simulink model "simulation_commande_adaptative_amine"  (R2020a)
settings: Solver=VariableStepAuto  StartTime=0.0  StopTime=100  RelTol=1e-3
settings Model: Creator=amine  LastModifiedBy=lenovo

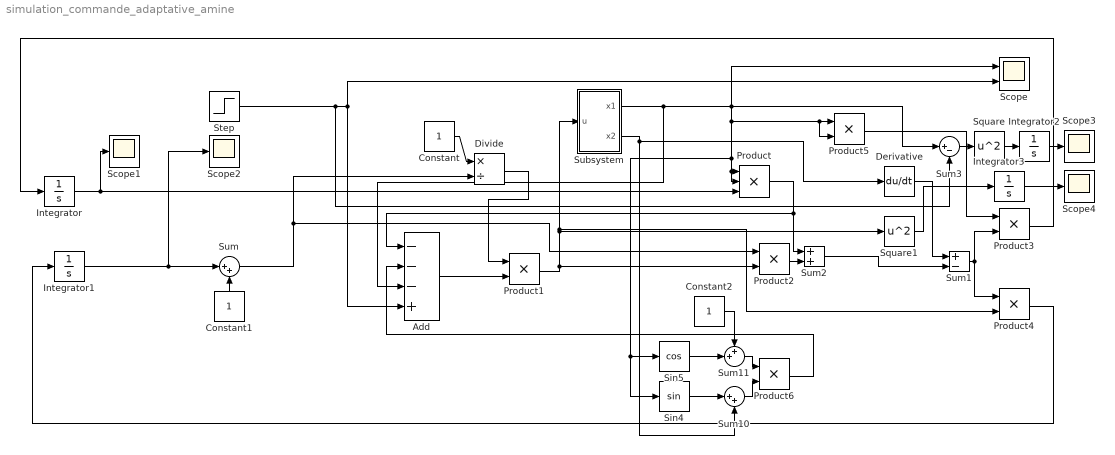
== system simulation_commande_adaptative_amine ==
  Add : Sum  Inputs=---+
  Constant : Constant
  Constant1 : Constant
  Constant2 : Constant
  Derivative : Derivative
  Divide : Product  Inputs=*/
  Integrator{,1..3} (4 alike) : Integrator
  Product : Product  Inputs=3
  Product{1..6} (6 alike) : Product
  Scope : Scope  NumInputPorts=2
  Scope{1..4} (4 alike) : Scope
  Sin4 : Trigonometry
  Sin5 : Trigonometry  Operator=cos
  Square : Math  Operator=square  SaturateOnIntegerOverflow=on
  Square1 : Math  Operator=square  SaturateOnIntegerOverflow=on
  Step : Step  Time=0  SampleTime=0
  Subsystem : Subsystem
  Sum : Sum  Inputs=|++
  Sum1 : Sum  Inputs=+-
  Sum10 : Sum  Inputs=|++
  Sum11 : Sum  Inputs=++|
  Sum2 : Sum
  Sum3 : Sum  Inputs=|+-
  wires:
  Sin5/1 -> Sum11/2
  Sum10/1 -> Product6/2
  Subsystem/2(x2) -> Derivative/1, Sum10/2
  Product/1 -> Sum2/1, Add/1
  Sin4/1 -> Sum10/1
  Product6/1 -> Add/2
  Constant2/1 -> Sum11/1
  Subsystem/1(x1) -> Add/3, Sum3/1, Product5/2, Product5/1, Product/2, Product/1, Sin5/1, Sin4/1, Scope/1
  Sum11/1 -> Product6/1
  Add/1 -> Product1/2
  Step/1 -> Sum3/2, Scope/2, Add/4
  Product1/1 -> Product2/2, Subsystem/1(u), Product4/2, Square1/1
  Constant/1 -> Divide/1
  Sum/1 -> Product2/1, Divide/2
  Constant1/1 -> Sum/2
  Integrator1/1 -> Scope2/1, Sum/1
  Divide/1 -> Product1/1
  Integrator/1 -> Scope1/1, Product/3
  Derivative/1 -> Sum1/1
  Product2/1 -> Sum2/2
  Sum2/1 -> Sum1/2
  Sum1/1 -> Product3/2, Product4/1
  Product5/1 -> Product3/1
  Product3/1 -> Integrator/1
  Product4/1 -> Integrator1/1
  Integrator2/1 -> Scope3/1
  Integrator3/1 -> Scope4/1
  Sum3/1 -> Square/1
  Square/1 -> Integrator2/1
  Square1/1 -> Integrator3/1

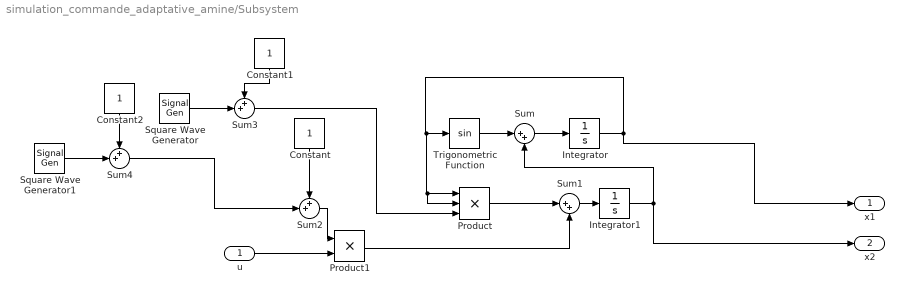
== system simulation_commande_adaptative_amine/Subsystem ==
  u : Inport
  Constant : Constant
  Constant1 : Constant
  Constant2 : Constant
  Integrator : Integrator
  Integrator1 : Integrator
  Product : Product  Inputs=3
  Product1 : Product
  Square Wave Generator : SignalGenerator  WaveForm=square  Amplitude=0.2  Frequency=0.05
  Square Wave Generator1 : SignalGenerator  WaveForm=square  Amplitude=0.2  Frequency=0.05
  Sum : Sum  Inputs=|++
  Sum1 : Sum  Inputs=|++
  Sum2 : Sum  Inputs=++|
  Sum3 : Sum  Inputs=++|
  Sum4 : Sum  Inputs=++|
  Trigonometric Function : Trigonometry
  x1 : Outport
  x2 : Outport  Port=2
  wires:
  Sum1/1 -> Integrator1/1
  Product/1 -> Sum1/1
  Integrator1/1 -> Sum/2, x2/1
  Trigonometric Function/1 -> Sum/1
  Integrator/1 -> Product/2, Product/1, Trigonometric Function/1, x1/1
  Sum/1 -> Integrator/1
  u/1 -> Product1/2
  Product1/1 -> Sum1/2
  Constant/1 -> Sum2/1
  Sum4/1 -> Sum2/2
  Sum2/1 -> Product1/1
  Square Wave Generator/1 -> Sum3/2
  Constant1/1 -> Sum3/1
  Sum3/1 -> Product/3
  Constant2/1 -> Sum4/1
  Square Wave Generator1/1 -> Sum4/2
